simulink model "AmpliSeguidorDeLinea"  (R2023b)
settings: Solver=FixedStepDiscrete  StartTime=0.0  StopTime=inf  FixedStep=0.01  RelTol=1e-3  EnableMultiTasking=on
model workspace (MAT data in the model file):
  baldosa = 0.48
  baldosa2 = 0.41
  d = 0.2625
libraries: slpidlib x1
settings Model: ExtModeTrigDuration=2  Creator=Usuario_UMA  LastModifiedBy=pablo
settings SolverCC: AlgebraicLoopSolver=TrustRegion  AutoInsertRateTranBlk=on
settings OptimizationCC: EnhancedBackFolding=on  PassReuseOutputArgsAs=Individual arguments  ZeroExternalMemoryAtStartup=off  ZeroInternalMemoryAtStartup=off  MaxStackSize=64  OptimizeBlockOrder=speed  DifferentSizesBufferReuse=on  EfficientTunableParamExpr=on
settings DebuggingCC: ParameterTunabilityLossMsg=error  UnconnectedInputMsg=warning  UnconnectedOutputMsg=warning  UnconnectedLineMsg=warning
settings HardwareCC: ProdBitPerInt=16  ProdBitPerPointer=16  ProdBitPerSizeT=16  ProdBitPerPtrDiffT=16  ProdLargestAtomicFloat=None  ProdWordSize=8  ProdHWDeviceType=Atmel->AVR  UseEmbeddedCoderFeatures=off  UseSimulinkCoderFeatures=off
settings ModelReferenceCC: EnableRefExpFcnMdlSchedulingChecks=on
settings SFSimCC: MATLABDynamicMemAlloc=off
settings RTWCC: Description=Embedded Coder  SystemTargetFile=ert.tlc  HardwareBoard=Arduino Mega 2560  TemplateMakefile=ert_default_tmf  Toolchain=Arduino AVR  BuildConfiguration=Faster Runs  DLArmComputeVersion=19.05
settings CodeAppCC: ForceParamTrailComments=on  IgnoreCustomStorageClasses=off  OperatorAnnotations=on  SimulinkDataObjDesc=on  SFDataObjDesc=on  MangleLength=10  InsertBlockDesc=on
settings ERTTargetCC: SupportContinuousTime=on  SupportNonInlinedSFcns=on  SupportVariableSizeSignals=on  ExtModeTransport=3  ExtModeStaticAlloc=on  ExtModeAutomaticAllocSize=off  ExtModeStaticAllocSize=2048  ExtModeMexFile=ext_xcp  ExtModeIntrfLevel=Level2 - Open

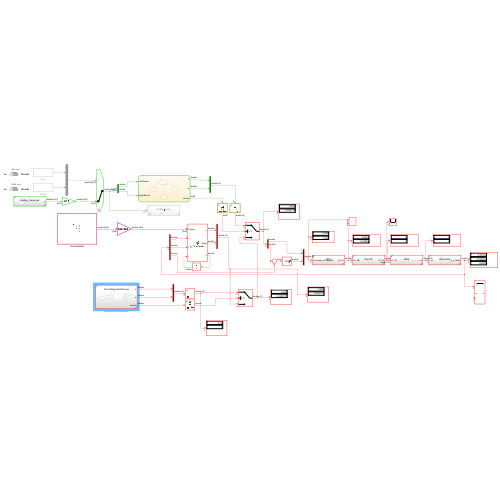
[thumbnail: Simulink's stored preview of the top-level diagram]
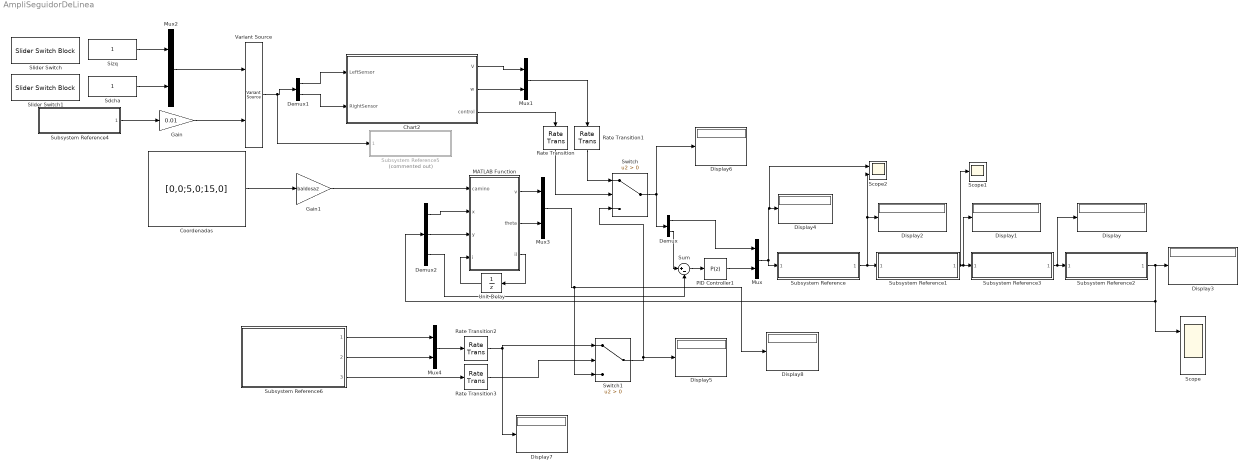
== system AmpliSeguidorDeLinea ==
  Chart2 : Stateflow chart  TreatAsAtomicUnit=on
  Coordenadas : Constant  Value=[0,0;5,0;15,0]
  Demux : Demux  Outputs=2
  Demux1 : Demux  Outputs=2
  Demux2 : Demux  Outputs=3
  Display{,1..8} (9 alike) : Display
  Gain : Gain  Gain=0.01  OutDataTypeStr=double
  Gain1 : Gain  Gain=baldosa2
  MATLAB Function : MATLAB Function  TreatAsAtomicUnit=on
  Mux{,1..4} (5 alike) : Mux  Inputs=2
  PID Controller1 : slpidlib/PID Controller  Controller=P  Form=Parallel  TimeDomain=Discrete-time  UseExternalTs=off  SampleTime=-1  IntegratorMethod=Forward Euler  FilterMethod=Forward Euler  ControllerParametersSource=internal  P=4.05578986502356  I=1  UseKiTs=off  D=0  N=100  UseFilter=on  TunerSelectOption=Transfer Function Based (PID Tuner App)  InitialConditionSource=internal  InitialConditionForIntegrator=0  InitialConditionForFilter=0  DifferentiatorICPrevScaledInput=0  ExternalReset=none  TrackingMode=off  Kt=1  LimitOutput=on  SatLimitsSource=internal  UpperSaturationLimit=1.5  LowerSaturationLimit=-1.5  LinearizeAsGain=on  AntiWindupMode=none  Kb=1  LimitIntegrator=off  UpperIntegratorSaturationLimit=inf  LowerIntegratorSaturationLimit=-inf  POutMin=[]  POutMax=[]  IOutMin=[]  IOutMax=[]  DOutMin=[]  DOutMax=[]  NOutMin=[]  NOutMax=[]  SumOutMin=[]  SumOutMax=[]  SaturationOutMin=[]  SaturationOutMax=[]  PParamMin=[]  PParamMax=[]  IParamMin=[]  IParamMax=[]  DParamMin=[]  DParamMax=[]  NParamMin=[]  NParamMax=[]  KbParamMin=[]  KbParamMax=[]  KtParamMin=[]  KtParamMax=[]  KbOutMin=[]  KbOutMax=[]  KtOutMin=[]  KtOutMax=[]  IntegratorOutMin=[]  IntegratorOutMax=[]  FilterOutMin=[]  FilterOutMax=[]  SumI1OutMin=[]  SumI1OutMax=[]  SumI2OutMin=[]  SumI2OutMax=[]  SumI3OutMin=[]  SumI3OutMax=[]  SumI4OutMin=[]  SumI4OutMax=[]  SumDOutMin=[]  SumDOutMax=[]  DifferentiatorOutMin=[]  DifferentiatorOutMax=[]  FilterDiffOutCoefMin=[]  FilterDiffOutCoefMax=[]  ReciprocalOutMin=[]  ReciprocalOutMax=[]  SumDenOutMin=[]  SumDenOutMax=[]  SumNumOutMin=[]  SumNumOutMax=[]  DivideOutMin=[]  DivideOutMax=[]  UdiffTsProdOutMin=[]  UdiffTsProdOutMax=[]  NTsProdOutMin=[]  NTsProdOutMax=[]  UintegralTsProdOutMin=[]  UintegralTsProdOutMax=[]  UngainTsProdOutMin=[]  UngainTsProdOutMax=[]  ClampingZeroOutDataTypeStr=Inherit: Inherit via back propagation  ClampingZeroOutMin=[]  ClampingZeroOutMax=[]  FilterDenConstantOutDataTypeStr=Inherit: Inherit via back propagation  FilterDenConstantOutMin=[]  FilterDenConstantOutMax=[]  PCopyOutDataTypeStr=Inherit: Inherit via back propagation  PCopyOutMin=[]  PCopyOutMax=[]  NCopyOutDataTypeStr=Inherit: Inherit via back propagation  NCopyOutMin=[]  NCopyOutMax=[]  IntegratorContinuousStateAttributes=''  IntegratorStateMustResolveToSignalObject=off  IntegratorRTWStateStorageClass=Auto  FilterContinuousStateAttributes=''  FilterStateMustResolveToSignalObject=off  FilterRTWStateStorageClass=Auto  ParallelPVariant=InternalParameters  IdealPVariant=Disabled  IVariant=Disabled  DVariant=Disabled  IntegratorVariant=Disabled  SatVariant=Enabled  AWVariant=Disabled  PCopyVariant=Disabled  TRVariant=Disabled  FdbkBlocksVariant=Forward  IdealPFdbkVariant=Disabled  SatFdbkVariant=Disabled  DerivativeFilterVariant=Disabled  NVariant=Disabled  NCopyVariant=Disabled_SignalSpec  FilterICVariant=Disabled  IntegratorICVariant=Disabled  ExternalResetVariant=Disabled  TRSumVariant=Passthrough  SumFdbkVariant=Disabled  SumVariant=Passthrough_P  TsampFilterVariant=InternalTs  TsampNgainVariant=Passthrough  TsampIntegralVariant=Disabled_SignalSpec  ExternalSaturationOutDataTypeStr=Inherit: Same as second input
  Rate Transition{,1..3} (4 alike) : RateTransition
  Scope : Scope  NumInputPorts=2
  Scope1 : Scope
  Scope2 : Scope  NumInputPorts=2
  Sdcha : Constant
  Sizq : Constant
  Slider Switch : SliderSwitchBlock
      settings: Values={{'Libre', 'Obstaculo'}, [1 0.29]}
  Slider Switch1 : SliderSwitchBlock
      settings: Values={{'Libre', 'Obstaculo'}, [1 0.29]}
  Subsystem Reference : Subsystem  ReferencedSubsystem=MCI
  Subsystem Reference1 : Subsystem  ReferencedSubsystem=PieroCV
  Subsystem Reference2 : Subsystem  ReferencedSubsystem=Odometria
  Subsystem Reference3 : Subsystem  ReferencedSubsystem=MCD
  Subsystem Reference4 : Subsystem  ReferencedSubsystem=Modelo_Sensores
  Subsystem Reference5 : Subsystem  Commented=on  ReferencedSubsystem=Modelo_Leds
  Subsystem Reference6 : Subsystem  ReferencedSubsystem=ContorlSeguidorDeLinea
  Sum : Sum  Inputs=|+-
  Switch : Switch  Criteria=u2 > Threshold  SaturateOnIntegerOverflow=off  InputSameDT=off
  Switch1 : Switch  Criteria=u2 > Threshold  SaturateOnIntegerOverflow=off  InputSameDT=off
  Unit Delay : UnitDelay  SampleTime=-1  HasFrameUpgradeWarning=on
  Variant Source : VariantSource  VariantControlMode=sim codegen switching
  wires:
  Subsystem Reference3/1 -> Subsystem Reference2/1, Display/1
  Subsystem Reference1/1 -> Scope1/1, Display1/1, Subsystem Reference3/1
  Subsystem Reference/1 -> Scope2/2, Display2/1, Subsystem Reference1/1
  Subsystem Reference2/1 -> Display3/1, Scope/1, Demux2/1
  Mux/1 -> Subsystem Reference/1, Scope2/1, Display4/1
  Sum/1 -> PID Controller1/1
  PID Controller1/1 -> Mux/2
  Demux2/3 -> Sum/2
  MATLAB Function/3(il) -> Unit Delay/1
  Unit Delay/1 -> MATLAB Function/4(i)
  Demux2/1 -> MATLAB Function/2(x)
  Demux2/2 -> MATLAB Function/3(y)
  Subsystem Reference4/1 -> Gain/1
  Chart2/3(control) -> Rate Transition/1
  Rate Transition1/1 -> Switch/1
  Sizq/1 -> Mux2/1
  Mux2/1 -> Variant Source/1
  Variant Source/1 -> Subsystem Reference5/1, Demux1/1
  Chart2/2(w) -> Mux1/2
  Sdcha/1 -> Mux2/2
  Demux1/1 -> Chart2/1(LeftSensor)
  Demux1/2 -> Chart2/2(RightSensor)
  Mux1/1 -> Rate Transition1/1
  Chart2/1(V) -> Mux1/1
  Rate Transition/1 -> Switch/2
  Gain/1 -> Variant Source/2
  MATLAB Function/1(v) -> Mux3/1
  MATLAB Function/2(theta) -> Mux3/2
  Mux3/1 -> Switch1/3, Display8/1
  Demux/2 -> Sum/1
  Demux/1 -> Mux/1
  Gain1/1 -> MATLAB Function/1(camino)
  Coordenadas/1 -> Gain1/1
  Subsystem Reference6/1 -> Mux4/1
  Subsystem Reference6/2 -> Mux4/2
  Mux4/1 -> Rate Transition2/1
  Subsystem Reference6/3 -> Rate Transition3/1
  Rate Transition2/1 -> Switch1/1, Display7/1
  Rate Transition3/1 -> Switch1/2
  Switch1/1 -> Switch/3, Display5/1
  Switch/1 -> Demux/1, Display6/1

== stateflow chart AmpliSeguidorDeLinea/Chart2 ==
  state SinObstaculos
    en:
    control = 0;
    V = 0.205;
    w = 0;
  state ObstaculoDcha
    en:
    control = 1;
    V = 0.1;
    w = 1;
  state ObstaculoIzq
    en:
    control = 1;
    V = 0.1;
    w = -1;
  state ObstaculoFrente
    en:
    control = 1;
    V = 0;
    w = 2;
  (default) -> SinObstaculos
  SinObstaculos -> ObstaculoDcha [order 2] : [RightSensor<0.3]
  SinObstaculos -> ObstaculoIzq [order 1] : [LeftSensor<0.3]
  ObstaculoIzq -> SinObstaculos [order 1] : after(3,sec)
  ObstaculoDcha -> SinObstaculos [order 1] : after(3,sec)
  ObstaculoFrente -> SinObstaculos : after(3,sec)
  ObstaculoIzq -> ObstaculoFrente [order 2] : [RightSensor<0.3]
  ObstaculoDcha -> ObstaculoFrente [order 2] : [LeftSensor<0.3]
  data: V output double size=1; w output double size=1; LeftSensor input size=1; RightSensor input size=1; control output uint8 size=1
  data V settings: description=Velocidad lineal del vehiculo

== matlab function AmpliSeguidorDeLinea/MATLAB Function ==
  data: camino input; v output; x input; y input; i input; theta output; il output
function [v,theta,il] = MyPurePerduit(camino,x,y,i)
L = 0.05; %Distancia de persecucion
v = 0.205;
i = i+1;
if length(camino)>i %Mientras haya camino
    %Calculamos distancia al objetivo
    distancia = sqrt((camino(i,1)-x)^2 + (camino(i,2)-y)^2);
    while(distancia<L)&&(length(camino)>i) %ya hemos
        i = i + 1; %Actualizar objetivo
        distancia = sqrt((camino(i,1)-x)^2 + (camino(i,2)-y)^2);
        v=0.205;
    end
    %Calculo de la orientacion al punto i-esimo
    theta = atan2((camino(i,2)-y),(camino(i,1)-x));
else %Si ha llegado al objetivo final se para
    theta = 0;
    v = 0;
end

if i<(length(camino))
    il = i -1;
else
    il = i;
end
end
